simulink model "CommSys_300_Bus_Area1_Part2"  (Simulink 8.0)
settings: Solver=ode45  StartTime=0.0  StopTime=3800  RelTol=1e-3
libraries: PiccSIM x79
settings Model: Creator=svenda  LastModifiedBy=svenda

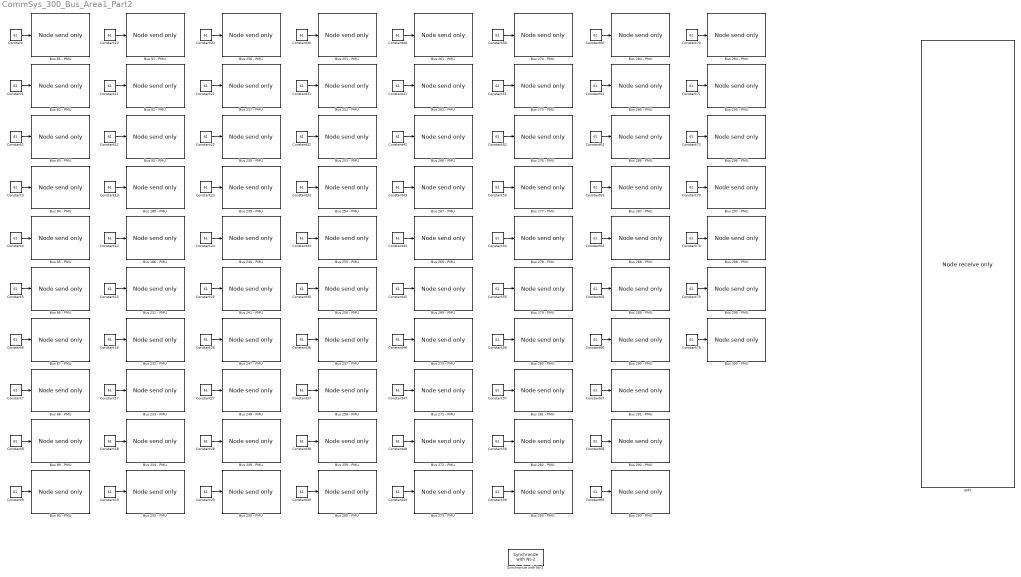
== system CommSys_300_Bus_Area1_Part2 ==
  Bus 180 - PMU : PiccSIM/Node send only  ID=13  time_or_seq=Timestamp  sendSchedule=Fixed sampling time  h=2  duty_cycle=1  sendEnable=off  pTypesSend=[113]  sendDataStructure={{'double'}}  externalID=off  sendID={[77]}  coordinates=[0, 0]  IP=NS2_IP
  Bus 186 - PMU : PiccSIM/Node send only  ID=14  time_or_seq=Timestamp  sendSchedule=Fixed sampling time  h=2  duty_cycle=1  sendEnable=off  pTypesSend=[114]  sendDataStructure={{'double'}}  externalID=off  sendID={[77]}  coordinates=[0, 0]  IP=NS2_IP
  Bus 231 - PMU : PiccSIM/Node send only  ID=15  time_or_seq=Timestamp  sendSchedule=Fixed sampling time  h=2  duty_cycle=1  sendEnable=off  pTypesSend=[115]  sendDataStructure={{'double'}}  externalID=off  sendID={[77]}  coordinates=[0, 0]  IP=NS2_IP
  Bus 232 - PMU : PiccSIM/Node send only  ID=16  time_or_seq=Timestamp  sendSchedule=Fixed sampling time  h=2  duty_cycle=1  sendEnable=off  pTypesSend=[116]  sendDataStructure={{'double'}}  externalID=off  sendID={[77]}  coordinates=[0, 0]  IP=NS2_IP
  Bus 233 - PMU : PiccSIM/Node send only  ID=17  time_or_seq=Timestamp  sendSchedule=Fixed sampling time  h=2  duty_cycle=1  sendEnable=off  pTypesSend=[117]  sendDataStructure={{'double'}}  externalID=off  sendID={[77]}  coordinates=[0, 0]  IP=NS2_IP
  Bus 234 - PMU : PiccSIM/Node send only  ID=18  time_or_seq=Timestamp  sendSchedule=Fixed sampling time  h=2  duty_cycle=1  sendEnable=off  pTypesSend=[118]  sendDataStructure={{'double'}}  externalID=off  sendID={[77]}  coordinates=[0, 0]  IP=NS2_IP
  Bus 235 - PMU : PiccSIM/Node send only  ID=19  time_or_seq=Timestamp  sendSchedule=Fixed sampling time  h=2  duty_cycle=1  sendEnable=off  pTypesSend=[119]  sendDataStructure={{'double'}}  externalID=off  sendID={[77]}  coordinates=[0, 0]  IP=NS2_IP
  Bus 236 - PMU : PiccSIM/Node send only  ID=20  time_or_seq=Timestamp  sendSchedule=Fixed sampling time  h=2  duty_cycle=1  sendEnable=off  pTypesSend=[120]  sendDataStructure={{'double'}}  externalID=off  sendID={[77]}  coordinates=[0, 0]  IP=NS2_IP
  Bus 237 - PMU : PiccSIM/Node send only  ID=21  time_or_seq=Timestamp  sendSchedule=Fixed sampling time  h=2  duty_cycle=1  sendEnable=off  pTypesSend=[121]  sendDataStructure={{'double'}}  externalID=off  sendID={[77]}  coordinates=[0, 0]  IP=NS2_IP
  Bus 238 - PMU : PiccSIM/Node send only  ID=22  time_or_seq=Timestamp  sendSchedule=Fixed sampling time  h=2  duty_cycle=1  sendEnable=off  pTypesSend=[122]  sendDataStructure={{'double'}}  externalID=off  sendID={[77]}  coordinates=[0, 0]  IP=NS2_IP
  Bus 239 - PMU : PiccSIM/Node send only  ID=23  time_or_seq=Timestamp  sendSchedule=Fixed sampling time  h=2  duty_cycle=1  sendEnable=off  pTypesSend=[123]  sendDataStructure={{'double'}}  externalID=off  sendID={[77]}  coordinates=[0, 0]  IP=NS2_IP
  Bus 240 - PMU : PiccSIM/Node send only  ID=24  time_or_seq=Timestamp  sendSchedule=Fixed sampling time  h=2  duty_cycle=1  sendEnable=off  pTypesSend=[124]  sendDataStructure={{'double'}}  externalID=off  sendID={[77]}  coordinates=[0, 0]  IP=NS2_IP
  Bus 241 - PMU : PiccSIM/Node send only  ID=25  time_or_seq=Timestamp  sendSchedule=Fixed sampling time  h=2  duty_cycle=1  sendEnable=off  pTypesSend=[125]  sendDataStructure={{'double'}}  externalID=off  sendID={[77]}  coordinates=[0, 0]  IP=NS2_IP
  Bus 247 - PMU : PiccSIM/Node send only  ID=26  time_or_seq=Timestamp  sendSchedule=Fixed sampling time  h=2  duty_cycle=1  sendEnable=off  pTypesSend=[126]  sendDataStructure={{'double'}}  externalID=off  sendID={[77]}  coordinates=[0, 0]  IP=NS2_IP
  Bus 248 - PMU : PiccSIM/Node send only  ID=27  time_or_seq=Timestamp  sendSchedule=Fixed sampling time  h=2  duty_cycle=1  sendEnable=off  pTypesSend=[127]  sendDataStructure={{'double'}}  externalID=off  sendID={[77]}  coordinates=[0, 0]  IP=NS2_IP
  Bus 249 - PMU : PiccSIM/Node send only  ID=28  time_or_seq=Timestamp  sendSchedule=Fixed sampling time  h=2  duty_cycle=1  sendEnable=off  pTypesSend=[128]  sendDataStructure={{'double'}}  externalID=off  sendID={[77]}  coordinates=[0, 0]  IP=NS2_IP
  Bus 250 - PMU : PiccSIM/Node send only  ID=29  time_or_seq=Timestamp  sendSchedule=Fixed sampling time  h=2  duty_cycle=1  sendEnable=off  pTypesSend=[129]  sendDataStructure={{'double'}}  externalID=off  sendID={[77]}  coordinates=[0, 0]  IP=NS2_IP
  Bus 251 - PMU : PiccSIM/Node send only  ID=30  time_or_seq=Timestamp  sendSchedule=Fixed sampling time  h=2  duty_cycle=1  sendEnable=off  pTypesSend=[130]  sendDataStructure={{'double'}}  externalID=off  sendID={[77]}  coordinates=[0, 0]  IP=NS2_IP
  Bus 252 - PMU : PiccSIM/Node send only  ID=31  time_or_seq=Timestamp  sendSchedule=Fixed sampling time  h=2  duty_cycle=1  sendEnable=off  pTypesSend=[131]  sendDataStructure={{'double'}}  externalID=off  sendID={[77]}  coordinates=[0, 0]  IP=NS2_IP
  Bus 253 - PMU : PiccSIM/Node send only  ID=32  time_or_seq=Timestamp  sendSchedule=Fixed sampling time  h=2  duty_cycle=1  sendEnable=off  pTypesSend=[132]  sendDataStructure={{'double'}}  externalID=off  sendID={[77]}  coordinates=[0, 0]  IP=NS2_IP
  Bus 254 - PMU : PiccSIM/Node send only  ID=33  time_or_seq=Timestamp  sendSchedule=Fixed sampling time  h=2  duty_cycle=1  sendEnable=off  pTypesSend=[133]  sendDataStructure={{'double'}}  externalID=off  sendID={[77]}  coordinates=[0, 0]  IP=NS2_IP
  Bus 255 - PMU : PiccSIM/Node send only  ID=34  time_or_seq=Timestamp  sendSchedule=Fixed sampling time  h=2  duty_cycle=1  sendEnable=off  pTypesSend=[134]  sendDataStructure={{'double'}}  externalID=off  sendID={[77]}  coordinates=[0, 0]  IP=NS2_IP
  Bus 256 - PMU : PiccSIM/Node send only  ID=35  time_or_seq=Timestamp  sendSchedule=Fixed sampling time  h=2  duty_cycle=1  sendEnable=off  pTypesSend=[135]  sendDataStructure={{'double'}}  externalID=off  sendID={[77]}  coordinates=[0, 0]  IP=NS2_IP
  Bus 257 - PMU : PiccSIM/Node send only  ID=36  time_or_seq=Timestamp  sendSchedule=Fixed sampling time  h=2  duty_cycle=1  sendEnable=off  pTypesSend=[136]  sendDataStructure={{'double'}}  externalID=off  sendID={[77]}  coordinates=[0, 0]  IP=NS2_IP
  Bus 258 - PMU : PiccSIM/Node send only  ID=37  time_or_seq=Timestamp  sendSchedule=Fixed sampling time  h=2  duty_cycle=1  sendEnable=off  pTypesSend=[137]  sendDataStructure={{'double'}}  externalID=off  sendID={[77]}  coordinates=[0, 0]  IP=NS2_IP
  Bus 259 - PMU : PiccSIM/Node send only  ID=38  time_or_seq=Timestamp  sendSchedule=Fixed sampling time  h=2  duty_cycle=1  sendEnable=off  pTypesSend=[138]  sendDataStructure={{'double'}}  externalID=off  sendID={[77]}  coordinates=[0, 0]  IP=NS2_IP
  Bus 260 - PMU : PiccSIM/Node send only  ID=39  time_or_seq=Timestamp  sendSchedule=Fixed sampling time  h=2  duty_cycle=1  sendEnable=off  pTypesSend=[139]  sendDataStructure={{'double'}}  externalID=off  sendID={[77]}  coordinates=[0, 0]  IP=NS2_IP
  Bus 261 - PMU : PiccSIM/Node send only  ID=40  time_or_seq=Timestamp  sendSchedule=Fixed sampling time  h=2  duty_cycle=1  sendEnable=off  pTypesSend=[140]  sendDataStructure={{'double'}}  externalID=off  sendID={[77]}  coordinates=[0, 0]  IP=NS2_IP
  Bus 262 - PMU : PiccSIM/Node send only  ID=41  time_or_seq=Timestamp  sendSchedule=Fixed sampling time  h=2  duty_cycle=1  sendEnable=off  pTypesSend=[141]  sendDataStructure={{'double'}}  externalID=off  sendID={[77]}  coordinates=[0, 0]  IP=NS2_IP
  Bus 266 - PMU : PiccSIM/Node send only  ID=42  time_or_seq=Timestamp  sendSchedule=Fixed sampling time  h=2  duty_cycle=1  sendEnable=off  pTypesSend=[142]  sendDataStructure={{'double'}}  externalID=off  sendID={[77]}  coordinates=[0, 0]  IP=NS2_IP
  Bus 267 - PMU : PiccSIM/Node send only  ID=43  time_or_seq=Timestamp  sendSchedule=Fixed sampling time  h=2  duty_cycle=1  sendEnable=off  pTypesSend=[143]  sendDataStructure={{'double'}}  externalID=off  sendID={[77]}  coordinates=[0, 0]  IP=NS2_IP
  Bus 268 - PMU : PiccSIM/Node send only  ID=44  time_or_seq=Timestamp  sendSchedule=Fixed sampling time  h=2  duty_cycle=1  sendEnable=off  pTypesSend=[144]  sendDataStructure={{'double'}}  externalID=off  sendID={[77]}  coordinates=[0, 0]  IP=NS2_IP
  Bus 269 - PMU : PiccSIM/Node send only  ID=45  time_or_seq=Timestamp  sendSchedule=Fixed sampling time  h=2  duty_cycle=1  sendEnable=off  pTypesSend=[145]  sendDataStructure={{'double'}}  externalID=off  sendID={[77]}  coordinates=[0, 0]  IP=NS2_IP
  Bus 270 - PMU : PiccSIM/Node send only  ID=46  time_or_seq=Timestamp  sendSchedule=Fixed sampling time  h=2  duty_cycle=1  sendEnable=off  pTypesSend=[146]  sendDataStructure={{'double'}}  externalID=off  sendID={[77]}  coordinates=[0, 0]  IP=NS2_IP
  Bus 271 - PMU : PiccSIM/Node send only  ID=47  time_or_seq=Timestamp  sendSchedule=Fixed sampling time  h=2  duty_cycle=1  sendEnable=off  pTypesSend=[147]  sendDataStructure={{'double'}}  externalID=off  sendID={[77]}  coordinates=[0, 0]  IP=NS2_IP
  Bus 272 - PMU : PiccSIM/Node send only  ID=48  time_or_seq=Timestamp  sendSchedule=Fixed sampling time  h=2  duty_cycle=1  sendEnable=off  pTypesSend=[148]  sendDataStructure={{'double'}}  externalID=off  sendID={[77]}  coordinates=[0, 0]  IP=NS2_IP
  Bus 273 - PMU : PiccSIM/Node send only  ID=49  time_or_seq=Timestamp  sendSchedule=Fixed sampling time  h=2  duty_cycle=1  sendEnable=off  pTypesSend=[149]  sendDataStructure={{'double'}}  externalID=off  sendID={[77]}  coordinates=[0, 0]  IP=NS2_IP
  Bus 274 - PMU : PiccSIM/Node send only  ID=50  time_or_seq=Timestamp  sendSchedule=Fixed sampling time  h=2  duty_cycle=1  sendEnable=off  pTypesSend=[150]  sendDataStructure={{'double'}}  externalID=off  sendID={[77]}  coordinates=[0, 0]  IP=NS2_IP
  Bus 275 - PMU : PiccSIM/Node send only  ID=51  time_or_seq=Timestamp  sendSchedule=Fixed sampling time  h=2  duty_cycle=1  sendEnable=off  pTypesSend=[151]  sendDataStructure={{'double'}}  externalID=off  sendID={[77]}  coordinates=[0, 0]  IP=NS2_IP
  Bus 276 - PMU : PiccSIM/Node send only  ID=52  time_or_seq=Timestamp  sendSchedule=Fixed sampling time  h=2  duty_cycle=1  sendEnable=off  pTypesSend=[152]  sendDataStructure={{'double'}}  externalID=off  sendID={[77]}  coordinates=[0, 0]  IP=NS2_IP
  Bus 277 - PMU : PiccSIM/Node send only  ID=53  time_or_seq=Timestamp  sendSchedule=Fixed sampling time  h=2  duty_cycle=1  sendEnable=off  pTypesSend=[153]  sendDataStructure={{'double'}}  externalID=off  sendID={[77]}  coordinates=[0, 0]  IP=NS2_IP
  Bus 278 - PMU : PiccSIM/Node send only  ID=54  time_or_seq=Timestamp  sendSchedule=Fixed sampling time  h=2  duty_cycle=1  sendEnable=off  pTypesSend=[154]  sendDataStructure={{'double'}}  externalID=off  sendID={[77]}  coordinates=[0, 0]  IP=NS2_IP
  Bus 279 - PMU : PiccSIM/Node send only  ID=55  time_or_seq=Timestamp  sendSchedule=Fixed sampling time  h=2  duty_cycle=1  sendEnable=off  pTypesSend=[155]  sendDataStructure={{'double'}}  externalID=off  sendID={[77]}  coordinates=[0, 0]  IP=NS2_IP
  Bus 280 - PMU : PiccSIM/Node send only  ID=56  time_or_seq=Timestamp  sendSchedule=Fixed sampling time  h=2  duty_cycle=1  sendEnable=off  pTypesSend=[156]  sendDataStructure={{'double'}}  externalID=off  sendID={[77]}  coordinates=[0, 0]  IP=NS2_IP
  Bus 281 - PMU : PiccSIM/Node send only  ID=57  time_or_seq=Timestamp  sendSchedule=Fixed sampling time  h=2  duty_cycle=1  sendEnable=off  pTypesSend=[157]  sendDataStructure={{'double'}}  externalID=off  sendID={[77]}  coordinates=[0, 0]  IP=NS2_IP
  Bus 282 - PMU : PiccSIM/Node send only  ID=58  time_or_seq=Timestamp  sendSchedule=Fixed sampling time  h=2  duty_cycle=1  sendEnable=off  pTypesSend=[158]  sendDataStructure={{'double'}}  externalID=off  sendID={[77]}  coordinates=[0, 0]  IP=NS2_IP
  Bus 283 - PMU : PiccSIM/Node send only  ID=59  time_or_seq=Timestamp  sendSchedule=Fixed sampling time  h=2  duty_cycle=1  sendEnable=off  pTypesSend=[159]  sendDataStructure={{'double'}}  externalID=off  sendID={[77]}  coordinates=[0, 0]  IP=NS2_IP
  Bus 284 - PMU : PiccSIM/Node send only  ID=60  time_or_seq=Timestamp  sendSchedule=Fixed sampling time  h=2  duty_cycle=1  sendEnable=off  pTypesSend=[160]  sendDataStructure={{'double'}}  externalID=off  sendID={[77]}  coordinates=[0, 0]  IP=NS2_IP
  Bus 285 - PMU : PiccSIM/Node send only  ID=61  time_or_seq=Timestamp  sendSchedule=Fixed sampling time  h=2  duty_cycle=1  sendEnable=off  pTypesSend=[161]  sendDataStructure={{'double'}}  externalID=off  sendID={[77]}  coordinates=[0, 0]  IP=NS2_IP
  Bus 286 - PMU : PiccSIM/Node send only  ID=62  time_or_seq=Timestamp  sendSchedule=Fixed sampling time  h=2  duty_cycle=1  sendEnable=off  pTypesSend=[162]  sendDataStructure={{'double'}}  externalID=off  sendID={[77]}  coordinates=[0, 0]  IP=NS2_IP
  Bus 287 - PMU : PiccSIM/Node send only  ID=63  time_or_seq=Timestamp  sendSchedule=Fixed sampling time  h=2  duty_cycle=1  sendEnable=off  pTypesSend=[163]  sendDataStructure={{'double'}}  externalID=off  sendID={[77]}  coordinates=[0, 0]  IP=NS2_IP
  Bus 288 - PMU : PiccSIM/Node send only  ID=64  time_or_seq=Timestamp  sendSchedule=Fixed sampling time  h=2  duty_cycle=1  sendEnable=off  pTypesSend=[164]  sendDataStructure={{'double'}}  externalID=off  sendID={[77]}  coordinates=[0, 0]  IP=NS2_IP
  Bus 289 - PMU : PiccSIM/Node send only  ID=65  time_or_seq=Timestamp  sendSchedule=Fixed sampling time  h=2  duty_cycle=1  sendEnable=off  pTypesSend=[165]  sendDataStructure={{'double'}}  externalID=off  sendID={[77]}  coordinates=[0, 0]  IP=NS2_IP
  Bus 290 - PMU : PiccSIM/Node send only  ID=66  time_or_seq=Timestamp  sendSchedule=Fixed sampling time  h=2  duty_cycle=1  sendEnable=off  pTypesSend=[166]  sendDataStructure={{'double'}}  externalID=off  sendID={[77]}  coordinates=[0, 0]  IP=NS2_IP
  Bus 291 - PMU : PiccSIM/Node send only  ID=67  time_or_seq=Timestamp  sendSchedule=Fixed sampling time  h=2  duty_cycle=1  sendEnable=off  pTypesSend=[167]  sendDataStructure={{'double'}}  externalID=off  sendID={[77]}  coordinates=[0, 0]  IP=NS2_IP
  Bus 292 - PMU : PiccSIM/Node send only  ID=68  time_or_seq=Timestamp  sendSchedule=Fixed sampling time  h=2  duty_cycle=1  sendEnable=off  pTypesSend=[168]  sendDataStructure={{'double'}}  externalID=off  sendID={[77]}  coordinates=[0, 0]  IP=NS2_IP
  Bus 293 - PMU : PiccSIM/Node send only  ID=69  time_or_seq=Timestamp  sendSchedule=Fixed sampling time  h=2  duty_cycle=1  sendEnable=off  pTypesSend=[169]  sendDataStructure={{'double'}}  externalID=off  sendID={[77]}  coordinates=[0, 0]  IP=NS2_IP
  Bus 294 - PMU : PiccSIM/Node send only  ID=70  time_or_seq=Timestamp  sendSchedule=Fixed sampling time  h=2  duty_cycle=1  sendEnable=off  pTypesSend=[170]  sendDataStructure={{'double'}}  externalID=off  sendID={[77]}  coordinates=[0, 0]  IP=NS2_IP
  Bus 295 - PMU : PiccSIM/Node send only  ID=71  time_or_seq=Timestamp  sendSchedule=Fixed sampling time  h=2  duty_cycle=1  sendEnable=off  pTypesSend=[171]  sendDataStructure={{'double'}}  externalID=off  sendID={[77]}  coordinates=[0, 0]  IP=NS2_IP
  Bus 296 - PMU : PiccSIM/Node send only  ID=72  time_or_seq=Timestamp  sendSchedule=Fixed sampling time  h=2  duty_cycle=1  sendEnable=off  pTypesSend=[172]  sendDataStructure={{'double'}}  externalID=off  sendID={[77]}  coordinates=[0, 0]  IP=NS2_IP
  Bus 297 - PMU : PiccSIM/Node send only  ID=73  time_or_seq=Timestamp  sendSchedule=Fixed sampling time  h=2  duty_cycle=1  sendEnable=off  pTypesSend=[173]  sendDataStructure={{'double'}}  externalID=off  sendID={[77]}  coordinates=[0, 0]  IP=NS2_IP
  Bus 298 - PMU : PiccSIM/Node send only  ID=74  time_or_seq=Timestamp  sendSchedule=Fixed sampling time  h=2  duty_cycle=1  sendEnable=off  pTypesSend=[174]  sendDataStructure={{'double'}}  externalID=off  sendID={[77]}  coordinates=[0, 0]  IP=NS2_IP
  Bus 299 - PMU : PiccSIM/Node send only  ID=75  time_or_seq=Timestamp  sendSchedule=Fixed sampling time  h=2  duty_cycle=1  sendEnable=off  pTypesSend=[175]  sendDataStructure={{'double'}}  externalID=off  sendID={[77]}  coordinates=[0, 0]  IP=NS2_IP
  Bus 300 - PMU : PiccSIM/Node send only  ID=76  time_or_seq=Timestamp  sendSchedule=Fixed sampling time  h=2  duty_cycle=1  sendEnable=off  pTypesSend=[176]  sendDataStructure={{'double'}}  externalID=off  sendID={[77]}  coordinates=[0, 0]  IP=NS2_IP
  Bus 81 - PMU : PiccSIM/Node send only  ID=0  time_or_seq=Timestamp  sendSchedule=Fixed sampling time  h=2  duty_cycle=1  sendEnable=off  pTypesSend=[10]  sendDataStructure={{'double'}}  externalID=off  sendID={[77]}  coordinates=[0, 0]  IP=NS2_IP
  Bus 82 - PMU : PiccSIM/Node send only  ID=1  time_or_seq=Timestamp  sendSchedule=Fixed sampling time  h=2  duty_cycle=1  sendEnable=off  pTypesSend=[11]  sendDataStructure={{'double'}}  externalID=off  sendID={[77]}  coordinates=[0, 0]  IP=NS2_IP
  Bus 83 - PMU : PiccSIM/Node send only  ID=2  time_or_seq=Timestamp  sendSchedule=Fixed sampling time  h=2  duty_cycle=1  sendEnable=off  pTypesSend=[12]  sendDataStructure={{'double'}}  externalID=off  sendID={[77]}  coordinates=[0, 0]  IP=NS2_IP
  Bus 84 - PMU : PiccSIM/Node send only  ID=3  time_or_seq=Timestamp  sendSchedule=Fixed sampling time  h=2  duty_cycle=1  sendEnable=off  pTypesSend=[13]  sendDataStructure={{'double'}}  externalID=off  sendID={[77]}  coordinates=[0, 0]  IP=NS2_IP
  Bus 85 - PMU : PiccSIM/Node send only  ID=4  time_or_seq=Timestamp  sendSchedule=Fixed sampling time  h=2  duty_cycle=1  sendEnable=off  pTypesSend=[14]  sendDataStructure={{'double'}}  externalID=off  sendID={[77]}  coordinates=[0, 0]  IP=NS2_IP
  Bus 86 - PMU : PiccSIM/Node send only  ID=5  time_or_seq=Timestamp  sendSchedule=Fixed sampling time  h=2  duty_cycle=1  sendEnable=off  pTypesSend=[15]  sendDataStructure={{'double'}}  externalID=off  sendID={[77]}  coordinates=[0, 0]  IP=NS2_IP
  Bus 87 - PMU : PiccSIM/Node send only  ID=6  time_or_seq=Timestamp  sendSchedule=Fixed sampling time  h=2  duty_cycle=1  sendEnable=off  pTypesSend=[16]  sendDataStructure={{'double'}}  externalID=off  sendID={[77]}  coordinates=[0, 0]  IP=NS2_IP
  Bus 88 - PMU : PiccSIM/Node send only  ID=7  time_or_seq=Timestamp  sendSchedule=Fixed sampling time  h=2  duty_cycle=1  sendEnable=off  pTypesSend=[17]  sendDataStructure={{'double'}}  externalID=off  sendID={[77]}  coordinates=[0, 0]  IP=NS2_IP
  Bus 89 - PMU : PiccSIM/Node send only  ID=8  time_or_seq=Timestamp  sendSchedule=Fixed sampling time  h=2  duty_cycle=1  sendEnable=off  pTypesSend=[18]  sendDataStructure={{'double'}}  externalID=off  sendID={[77]}  coordinates=[0, 0]  IP=NS2_IP
  Bus 90 - PMU : PiccSIM/Node send only  ID=9  time_or_seq=Timestamp  sendSchedule=Fixed sampling time  h=2  duty_cycle=1  sendEnable=off  pTypesSend=[19]  sendDataStructure={{'double'}}  externalID=off  sendID={[77]}  coordinates=[0, 0]  IP=NS2_IP
  Bus 91 - PMU : PiccSIM/Node send only  ID=10  time_or_seq=Timestamp  sendSchedule=Fixed sampling time  h=2  duty_cycle=1  sendEnable=off  pTypesSend=[110]  sendDataStructure={{'double'}}  externalID=off  sendID={[77]}  coordinates=[0, 0]  IP=NS2_IP
  Bus 92 - PMU : PiccSIM/Node send only  ID=11  time_or_seq=Timestamp  sendSchedule=Fixed sampling time  h=2  duty_cycle=1  sendEnable=off  pTypesSend=[111]  sendDataStructure={{'double'}}  externalID=off  sendID={[77]}  coordinates=[0, 0]  IP=NS2_IP
  Bus 93 - PMU : PiccSIM/Node send only  ID=12  time_or_seq=Timestamp  sendSchedule=Fixed sampling time  h=2  duty_cycle=1  sendEnable=off  pTypesSend=[112]  sendDataStructure={{'double'}}  externalID=off  sendID={[77]}  coordinates=[0, 0]  IP=NS2_IP
  Constant{,1..76} (77 alike) : Constant  Value=61
  EMS : PiccSIM/Node receive only  ID=77  pTypes=[10, 11, 12, 13, 14, 15, 16, 17, 18, 19, 110, 111, 112, 113, 114, 115, 116, 117, 118, 119, 120, 121, 122, 123, 124, 125, 126, 127, 128, 129, 130, 131, 132, 133, 134, 135, 136, 137, 138, 139, 140, 141, 142, 143, 144, 145, 146, 147, 148, 149, 150, 151, 152, 153, 154, 155, 156, 157, 158, 159, 160, 161, 162, 163, 164, 165, 166, 167, 168, 169, 170, 171, 172, 173, 174, 175, 176]  receiveDataLengths={{[1]}, {[1]}, {[1]}, {[1]}, {[1]}, {[1]}, {[1]}, {[1]}, {[1]}, {[1]},{[1]}, {[1]}, {[1]}, {[1]}, {[1]}, {[1]}, {[1]}, {[1]}, {[1]}, {[1]},{[1]}, {[1]}, {[1]}, {[1]}, {[1]}, {[1]}, {[1]}, {[1]}, {[1]}, {[1]},{[1]}, {[1]}, {[1]}, {[1]}, {[1]}, {[1]}, {[1]}, {[1]}, {[1]}, {[1]},{[1]}, {[1]}, {[1]}, {[1]}, {[1]}, {[1]}, {[1]}, {[1]}, {[1]}, {[1]},{[1]}, {[1]}, {[1]}, {[1]}, {[1]}, {[1]}, {[1]}, {[1]}, {[1]}, {[1]},{[1]}, {[1]}, {[1]}, {[1]}, {[1]}, {[1]}, {[1]}, {[1]}, {[1]}, {[1]},{[1]}, {[1]}, {[1]}, {[1]}, {[1]}, {[1]}, {[1]}}  receiveDataStructure={{'double'}, {'double'}, {'double'}, {'double'}, {'double'}, {'double'}, {'double'}, {'double'}, {'double'}, {'double'},{'double'}, {'double'}, {'double'}, {'double'}, {'double'}, {'double'}, {'double'}, {'double'}, {'double'}, {'double'},{'double'}, {'double'}, {'double'}, {'double'}, {'double'}, {'double'}, {'double'}, {'double'}, {'double'}, {'double'},{'double'}, {'double'}, {'double'}, {'double'}, {'double'}, {'double'}, {'double'}, {'double'}, {'double'}, {'double'},{'double'}, {'double'}, {'double'}, {'double'}, {'double'}, {'double'}, {'double'}, {'double'}, {'double'}, {'double'},{'double'}, {'double'}, {'double'}, {'double'}, {'double'}, {'double'}, {'double'}, {'double'}, {'double'}, {'double'},{'double'}, {'double'}, {'double'}, {'double'}, {'double'}, {'double'}, {'double'}, {'double'}, {'double'}, {'double'},{'double'}, {'double'}, {'double'}, {'double'}, {'double'}, {'double'}, {'double'}}  recFrom={[0], [1], [2], [3], [4], [5], [6], [7], [8], [9], [10], [11], [12], [13], [14], [15], [16], [17], [18], [19], [20], [21], [22], [23], [24], [25], [26], [27], [28], [29], [30], [31], [32], [33], [34], [35], [36], [37], [38], [39], [40], [41], [42], [43], [44], [45], [46], [47], [48], [49], [50], [51], [52], [53], [54], [55], [56], [57], [58], [59], [60], [61], [62], [63], [64], [65], [66], [67], [68], [69], [70], [71], [72], [73], [74], [75], [76]}  coordinates=[0, 0]  IP=NS2_IP
  Synchronize with Ns-2 : PiccSIM/Synchronize with Ns-2  Priority=100000  c=1  port=23201  IP=NS2_IP
  wires:
  Constant/1 -> Bus 81 - PMU/1
  Constant1/1 -> Bus 82 - PMU/1
  Constant2/1 -> Bus 83 - PMU/1
  Constant3/1 -> Bus 84 - PMU/1
  Constant4/1 -> Bus 85 - PMU/1
  Constant5/1 -> Bus 86 - PMU/1
  Constant6/1 -> Bus 87 - PMU/1
  Constant7/1 -> Bus 88 - PMU/1
  Constant8/1 -> Bus 89 - PMU/1
  Constant9/1 -> Bus 90 - PMU/1
  Constant10/1 -> Bus 91 - PMU/1
  Constant11/1 -> Bus 92 - PMU/1
  Constant12/1 -> Bus 93 - PMU/1
  Constant13/1 -> Bus 180 - PMU/1
  Constant14/1 -> Bus 186 - PMU/1
  Constant15/1 -> Bus 231 - PMU/1
  Constant16/1 -> Bus 232 - PMU/1
  Constant17/1 -> Bus 233 - PMU/1
  Constant18/1 -> Bus 234 - PMU/1
  Constant19/1 -> Bus 235 - PMU/1
  Constant20/1 -> Bus 236 - PMU/1
  Constant21/1 -> Bus 237 - PMU/1
  Constant22/1 -> Bus 238 - PMU/1
  Constant23/1 -> Bus 239 - PMU/1
  Constant24/1 -> Bus 240 - PMU/1
  Constant25/1 -> Bus 241 - PMU/1
  Constant26/1 -> Bus 247 - PMU/1
  Constant27/1 -> Bus 248 - PMU/1
  Constant28/1 -> Bus 249 - PMU/1
  Constant29/1 -> Bus 250 - PMU/1
  Constant30/1 -> Bus 251 - PMU/1
  Constant31/1 -> Bus 252 - PMU/1
  Constant32/1 -> Bus 253 - PMU/1
  Constant33/1 -> Bus 254 - PMU/1
  Constant34/1 -> Bus 255 - PMU/1
  Constant35/1 -> Bus 256 - PMU/1
  Constant36/1 -> Bus 257 - PMU/1
  Constant37/1 -> Bus 258 - PMU/1
  Constant38/1 -> Bus 259 - PMU/1
  Constant39/1 -> Bus 260 - PMU/1
  Constant40/1 -> Bus 261 - PMU/1
  Constant41/1 -> Bus 262 - PMU/1
  Constant42/1 -> Bus 266 - PMU/1
  Constant43/1 -> Bus 267 - PMU/1
  Constant44/1 -> Bus 268 - PMU/1
  Constant45/1 -> Bus 269 - PMU/1
  Constant46/1 -> Bus 270 - PMU/1
  Constant47/1 -> Bus 271 - PMU/1
  Constant48/1 -> Bus 272 - PMU/1
  Constant49/1 -> Bus 273 - PMU/1
  Constant50/1 -> Bus 274 - PMU/1
  Constant51/1 -> Bus 275 - PMU/1
  Constant52/1 -> Bus 276 - PMU/1
  Constant53/1 -> Bus 277 - PMU/1
  Constant54/1 -> Bus 278 - PMU/1
  Constant55/1 -> Bus 279 - PMU/1
  Constant56/1 -> Bus 280 - PMU/1
  Constant57/1 -> Bus 281 - PMU/1
  Constant58/1 -> Bus 282 - PMU/1
  Constant59/1 -> Bus 283 - PMU/1
  Constant60/1 -> Bus 284 - PMU/1
  Constant61/1 -> Bus 285 - PMU/1
  Constant62/1 -> Bus 286 - PMU/1
  Constant63/1 -> Bus 287 - PMU/1
  Constant64/1 -> Bus 288 - PMU/1
  Constant65/1 -> Bus 289 - PMU/1
  Constant66/1 -> Bus 290 - PMU/1
  Constant67/1 -> Bus 291 - PMU/1
  Constant68/1 -> Bus 292 - PMU/1
  Constant69/1 -> Bus 293 - PMU/1
  Constant70/1 -> Bus 294 - PMU/1
  Constant71/1 -> Bus 295 - PMU/1
  Constant72/1 -> Bus 296 - PMU/1
  Constant73/1 -> Bus 297 - PMU/1
  Constant74/1 -> Bus 298 - PMU/1
  Constant75/1 -> Bus 299 - PMU/1
  Constant76/1 -> Bus 300 - PMU/1
